simulink model "curr_against_torques"  (R2017b)
settings: Solver=FixedStepAuto  StartTime=0.0  StopTime=inf  FixedStep=samp_time  RelTol=1e-3
InitFcn:
  | samp_time = 0.01
libraries: robotlib x10
settings Model: Creator=exo-hand  LastModifiedBy=exo-hand

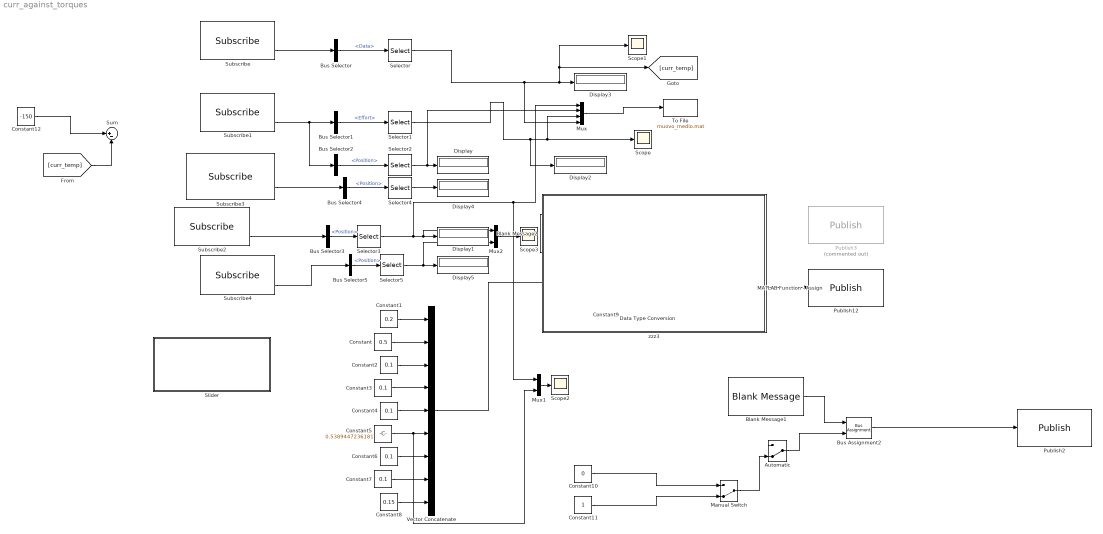
== system curr_against_torques ==
  "Automatic " : ManualSwitch  CurrentSetting=0
  Blank Message1 : robotlib/Blank Message  SourceLibraryInfo=This block requires Robotics System Toolbox  messageType=std_msgs/Bool  SampleTime=samp_time
      settings: SourceProductBaseCode=RO
  Blank Message2 : robotlib/Blank Message  SourceLibraryInfo=This block requires Robotics System Toolbox  messageType=sensor_msgs/JointState  SampleTime=samp_time
      settings: SourceProductBaseCode=RO
  Bus Assignment2 : BusAssignment  AssignedSignals=Data
  Bus Selector : BusSelector  OutputSignals=Data
  Bus Selector1 : BusSelector  OutputSignals=Effort
  Bus Selector{2..5} (4 alike) : BusSelector  OutputSignals=Position
  Constant : Constant  Value=0.5
  Constant1 : Constant  Value=0.2
  Constant10 : Constant  Value=0  OutDataTypeStr=boolean
  Constant11 : Constant  OutDataTypeStr=boolean
  Constant12 : Constant  Value=-150
  Constant{2..4,6..7} (5 alike) : Constant  Value=0.1
  Constant5 : Constant  Value=0.5389447236181
  Constant8 : Constant  Value=0.15
  Constant9 : Constant  Value=0
  Data Type Conversion : DataTypeConversion  OutDataTypeStr=uint32
  Display{,1..5} (6 alike) : Display
  MATLAB Function - Assign : MATLAB Function  TreatAsAtomicUnit=on
  Manual Switch : ManualSwitch  CurrentSetting=0
  Mux : Mux
  Mux1 : Mux  Inputs=2
  Mux2 : Mux  Inputs=2
  Publish12 : robotlib/Publish  SourceLibraryInfo=This block requires Robotics System Toolbox  topicSource=Select from ROS network  topic=/scan  messageType=sensor_msgs/JointState  messageQueueLength=1
      settings: SourceProductBaseCode=RO
  Publish2 : robotlib/Publish  SourceLibraryInfo=This block requires Robotics System Toolbox  topicSource=Specify your own  topic=/trigger_exo_hand  messageType=std_msgs/Bool  messageQueueLength=1
      settings: SourceProductBaseCode=RO
  Publish3 : robotlib/Publish  Commented=on  SourceLibraryInfo=This block requires Robotics System Toolbox  topicSource=Select from ROS network  topic=/joint_commands  messageType=plot_msgs/JointCommand  messageQueueLength=1
      settings: SourceProductBaseCode=RO
  Scope{,1..3} (4 alike) : Scope
  Selector{,1..2,4..5} (5 alike) : Selector  IndexOptions=Index vector (dialog)  Indices=6  OutputSizes=1
  Selector3 : Selector  IndexOptions=Index vector (dialog)  Indices=7  OutputSizes=1
  Slider : Subsystem  DialogController=hmiCreateDDGDialog  IsWebBlock=on  mask(MWDashboardBlock){webBlockId=65998c15-e69a-4696-9705-d828fcb41c7c, webBlockType=slider, ShowInLibBrowser=on, ShowInitialText=on, HMISrcModelName=curr_against_torques}
      mask prompts: webBlockId "WebBlock Id"; webBlockType "WebBlock Type"; HMISrcModelName "Source Model"
      mask help: SimulinkHMI:dialogs:SliderDialogDesc
      mask Help: helpview([docroot '/mapfiles/simulink.map'], 'hmi_slider')
      mask Display:
      | if strcmp(get_param(bdroot(gcb),'BlockDiagramType'), 'library')
      |     image([(matlabroot) '/toolbox/simulink/hmi/icons/Slider.png']);
      | end
  Subscribe : robotlib/Subscribe  SourceLibraryInfo=This block requires Robotics System Toolbox  topicSource=Select from ROS network  topic=/svh_controller/channel_currents  messageType=std_msgs/Float64MultiArray  sampleTime=samp_time  messageQueueLength=1
      settings: SourceProductBaseCode=RO
  Subscribe1 : robotlib/Subscribe  SourceLibraryInfo=This block requires Robotics System Toolbox  topicSource=Select from ROS network  topic=/svh_controller/channel_feedback  messageType=sensor_msgs/JointState  sampleTime=samp_time  messageQueueLength=1
      settings: SourceProductBaseCode=RO
  Subscribe2 : robotlib/Subscribe  SourceLibraryInfo=This block requires Robotics System Toolbox  topicSource=Select from ROS network  topic=/svh_controller/channel_targets  messageType=sensor_msgs/JointState  sampleTime=samp_time  messageQueueLength=1
      settings: SourceProductBaseCode=RO
  Subscribe3 : robotlib/Subscribe  SourceLibraryInfo=This block requires Robotics System Toolbox  topicSource=Select from ROS network  topic=/ur10_schunk/joint_states  messageType=sensor_msgs/JointState  sampleTime=0.01  messageQueueLength=1
      settings: SourceProductBaseCode=RO
  Subscribe4 : robotlib/Subscribe  SourceLibraryInfo=This block requires Robotics System Toolbox  topicSource=Select from ROS network  topic=/scan  messageType=sensor_msgs/JointState  sampleTime=samp_time  messageQueueLength=1
      settings: SourceProductBaseCode=RO
  Sum : Sum  Inputs=|+-
  To File : ToFile  Filename=muovo_medio.mat  MatrixName=serie
  Vector Concatenate : Concatenate  NumInputs=9
  zzz3 : Subsystem  TreatAsAtomicUnit=on
      settings: OpenFcn=% no-op
      mask Display: disp('')
  wires:
  Subscribe/2 -> Bus Selector/1
  Subscribe1/2 -> Bus Selector2/1, Bus Selector1/1
  Bus Selector/1 -> Selector/1  "<Data>"
  Selector/1 -> Mux/4, Display3/1, [curr_temp], Scope1/1
  Bus Selector1/1 -> Selector1/1  "<Effort>"
  Selector1/1 -> Display2/1, Mux/3, Scope/1
  Bus Selector2/1 -> Selector2/1  "<Position>"
  Selector2/1 -> Mux/2, Display/1
  Subscribe2/2 -> Bus Selector3/1
  Selector3/1 -> Mux1/1, Mux/1, Mux2/1, Display1/1
  Bus Selector3/1 -> Selector3/1  "<Position>"
  Constant9/1 -> Data Type Conversion/1
  Vector Concatenate/1 -> MATLAB Function - Assign/2(u)
  Data Type Conversion/1 -> MATLAB Function - Assign/3(timeStamp)
  Blank Message2/1 -> MATLAB Function - Assign/1(blankMessage)
  MATLAB Function - Assign/1(msg) -> Publish12/1
  Constant1/1 -> Vector Concatenate/1
  Constant/1 -> Vector Concatenate/2
  Constant2/1 -> Vector Concatenate/3
  Constant3/1 -> Vector Concatenate/4
  Constant4/1 -> Vector Concatenate/5
  Constant5/1 -> Mux1/2, Vector Concatenate/6
  Constant6/1 -> Vector Concatenate/7
  Constant7/1 -> Vector Concatenate/8
  Constant8/1 -> Vector Concatenate/9
  Mux/1 -> To File/1
  Constant10/1 -> Manual Switch/1
  Bus Assignment2/1 -> Publish2/1
  Constant11/1 -> Manual Switch/2
  Blank Message1/1 -> Bus Assignment2/1
  Manual Switch/1 -> "Automatic "/2
  "Automatic "/1 -> Bus Assignment2/2
  [curr_temp] -> Sum/2
  Constant12/1 -> Sum/1
  Mux1/1 -> Scope2/1
  Subscribe3/2 -> Bus Selector4/1
  Bus Selector4/1 -> Selector4/1  "<Position>"
  Selector4/1 -> Display4/1
  Selector5/1 -> Mux2/2, Display5/1
  Bus Selector5/1 -> Selector5/1  "<Position>"
  Subscribe4/2 -> Bus Selector5/1
  Mux2/1 -> Scope3/1

== system curr_against_torques/Slider ==

== system curr_against_torques/zzz3 ==

== matlab function curr_against_torques/MATLAB Function - Assign ==
  data: blankMessage input; u input; msg output Bus: SL_Bus_curr_against_torques_sensor_msgs_JointState; timeStamp input
function msg = assignArray(blankMessage,u,timeStamp)
%#codegen

% To set datatype of MSG output:
%  1. Create buses for this model: robotics.ros.createSimulinkBus(gcs)
%  1. Click "Edit Data" in  Toolstrip to open "Ports and Data Manager"
%  2. Select MSG and set datatype to "Bus: SL_Bus_<modelname>_<messageType>"
% See: 
% http://www.mathworks.com/help/simulink/ug/create-structures-in-matlab-function-blocks.html

% blankMessage (sensor_msgs/LaserScan) consists of 
%             Header: [1x1 Header]
%           AngleMin: 0
%           AngleMax: 0
%     AngleIncrement: 0
%      TimeIncrement: 0
%           ScanTime: 0
%           RangeMin: 0
%           RangeMax: 0
%             Ranges: [0x1 single]
%        Intensities: [0x1 single]

% Set Ranges array to have length 10, and modify indices 1, 3, 5 and 7
blankMessage.Header.Seq = timeStamp;
blankMessage.Position_SL_Info.CurrentLength = uint32(9); 
blankMessage.Position([1 2 3 4 5 6 7 8 9]) = [u(1) u(2) u(3) u(4) u(5) u(6) u(7) u(8) u(9)];
blankMessage.Velocity_SL_Info.CurrentLength = uint32(9); 
blankMessage.Velocity([1 2 3 4 5 6 7 8 9]) = zeros(1,9);
blankMessage.Effort_SL_Info.CurrentLength = uint32(9); 
blankMessage.Effort([1 2 3 4 5 6 7 8 9]) = zeros(1,9);
%blankMessage.Name.Data_SL_Info.CurrentLength = uint32(9);
%blankMessage.Name.Data([1 2 3 4 5 6 7 8 9]) = ['right_hand_Thumb_Flexion', 'right_hand_Thumb_Opposition', ...
%     'right_hand_Index_Finger_Distal','right_hand_Index_Finger_Proximal','right_hand_Middle_Finger_Distal','right_hand_Middle_Finger_Proximal',...
%     'right_hand_Ring_Finger','right_hand_Pinky','right_hand_index_spread'];

strArrayToAssign = {'right_hand_Thumb_Flexion', 'right_hand_Thumb_Opposition', ...
    'right_hand_Index_Finger_Distal','right_hand_Index_Finger_Proximal','right_hand_Middle_Finger_Distal','right_hand_Middle_Finger_Proximal',...
    'right_hand_Ring_Finger','right_hand_Pinky','right_hand_Finger_Spread'};


% Set the number of strings in the string array.
% msg (sensor_msgs/JointState) includes the following fields
%           Name : array of std_msgs/String (string array)
%   Name_SL_Info : struct with fields CurrentLength, ReceivedLength
numStringsInArray = length(strArrayToAssign);
blankMessage.Name_SL_Info.CurrentLength = uint32(numStringsInArray);

% Set the individual strings in the array
for idx=1:numStringsInArray
    str = strArrayToAssign{idx};
    strLength = length(str);
    blankMessage.Name(idx).Data(1:strLength) = uint8(str);
    blankMessage.Name(idx).Data_SL_Info.CurrentLength = uint32(strLength);
end
msg = blankMessage;
